simulink model "trigger"  (Simulink 7.9)
settings: Solver=ode45  StartTime=0.0  StopTime=10.0  RelTol=1e-3
settings Model: Creator=jdenil  LastModifiedBy=jdenil

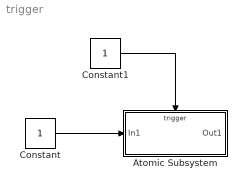
== system trigger ==
  Atomic Subsystem : Subsystem  TreatAsAtomicUnit=on
  Constant : Constant
  Constant1 : Constant
  wires:
  Constant/1 -> Atomic Subsystem/1(In1)
  Constant1/1 -> Atomic Subsystem/Trigger

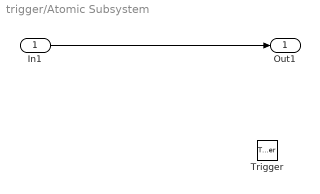
== system trigger/Atomic Subsystem ==
  In1 : Inport
  Trigger : TriggerPort  PortDimensions=1
  Out1 : Outport
  wires:
  In1/1 -> Out1/1
